simulink model "AckermanSimu"  (R2022a)
settings: Solver=VariableStepAuto  StartTime=0.0  StopTime=100  RelTol=1e-3
values from neighbouring files (symbols this model uses):
  a1 = 0.178    [param_tanques.m]
  A1 = 15.518    [param_tanques.m]
  A2 = A1 + 3e-5    (= 15.51803)    [param_tanques.m]
  a2 = a1+5e-5    (= 0.17805)    [param_tanques.m]
  g = 981    [param_tanques.m]
  K1 = K(1)    [Ackerman.m]    (also in param_tanques.m)
  K2 = [K(2) K(3)]    [Ackerman.m]    (also in param_tanques.m)
  Km = 4.6    [param_tanques.m]
  L0 = [0;0]    [param_tanques.m]
settings Model: Creator=joaom  LastModifiedBy=joaom

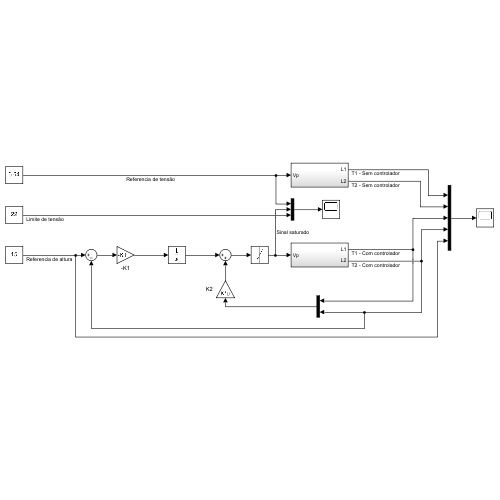
[thumbnail: Simulink's stored preview of the top-level diagram]
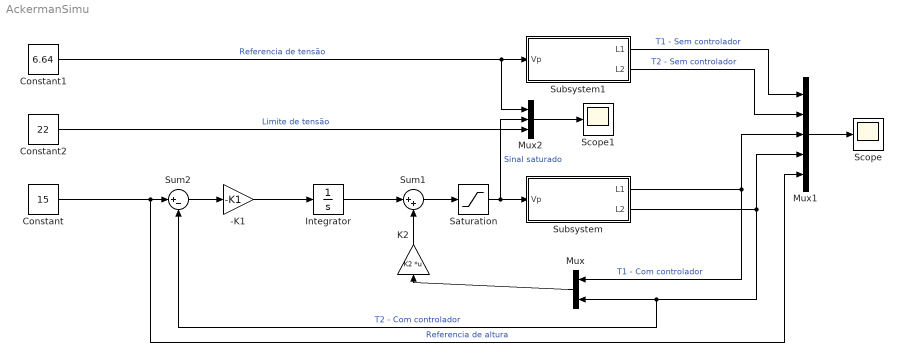
== system AckermanSimu ==
  -K1 : Gain  Gain=-K1
  Constant : Constant  Value=15
  Constant1 : Constant  Value=6.64
  Constant2 : Constant  Value=22
  Integrator : Integrator
  K2 : Gain  Gain=K2  Multiplication=Matrix(K*u)
  Mux : Mux  Inputs=2
  Mux1 : Mux  Inputs=5
  Mux2 : Mux  Inputs=3
  Saturation : Saturate  UpperLimit=22  LowerLimit=-22
  Scope : Scope
  Scope1 : Scope
  Subsystem : Subsystem
  Subsystem1 : Subsystem
  Sum1 : Sum  Inputs=|++
  Sum2 : Sum  Inputs=|+-
  wires:
  Constant/1 -> Mux1/5, Sum2/1  "Referencia de altura"
  Sum2/1 -> -K1/1
  -K1/1 -> Integrator/1
  Integrator/1 -> Sum1/1
  K2/1 -> Sum1/2
  Mux/1 -> K2/1
  Subsystem/2(L2) -> Mux1/4, Sum2/2, Mux/2  "T2 - Com controlador"
  Subsystem/1(L1) -> Mux1/3, Mux/1  "T1 - Com controlador"
  Mux1/1 -> Scope/1
  Constant1/1 -> Mux2/1, Subsystem1/1(Vp)  "Referencia de tensão"
  Subsystem1/1(L1) -> Mux1/1  "T1 - Sem controlador"
  Subsystem1/2(L2) -> Mux1/2  "T2 - Sem controlador"
  Mux2/1 -> Scope1/1
  Saturation/1 -> Mux2/2, Subsystem/1(Vp)  "Sinal saturado"
  Sum1/1 -> Saturation/1
  Constant2/1 -> Mux2/3  "Limite de tensão"

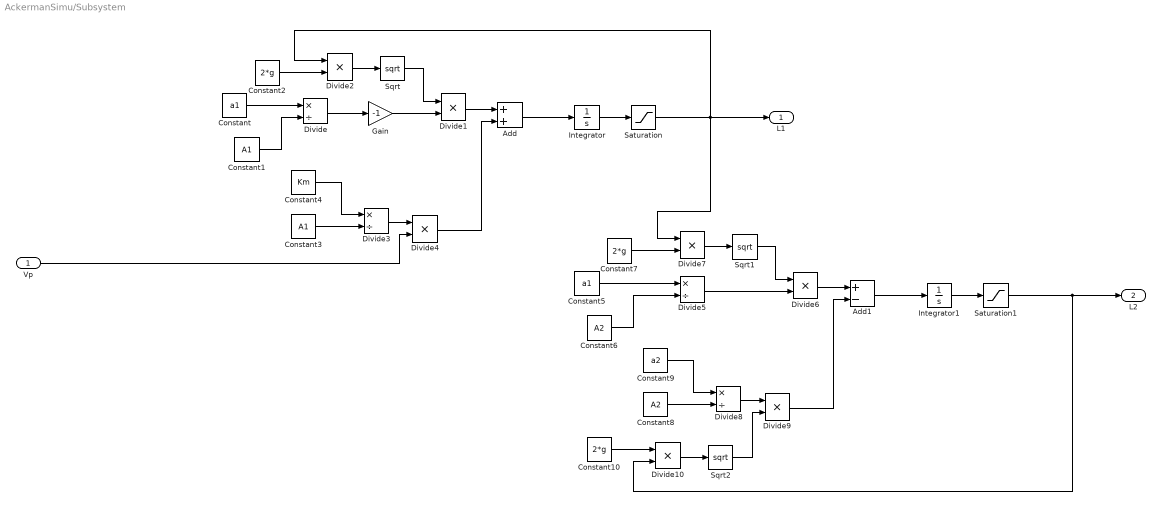
== system AckermanSimu/Subsystem ==
  Vp : Inport
  Add : Sum
  Add1 : Sum  Inputs=+-
  Constant : Constant  Value=a1
  Constant1 : Constant  Value=A1
  Constant10 : Constant  Value=2*g
  Constant2 : Constant  Value=2*g
  Constant3 : Constant  Value=A1
  Constant4 : Constant  Value=Km
  Constant5 : Constant  Value=a1
  Constant6 : Constant  Value=A2
  Constant7 : Constant  Value=2*g
  Constant8 : Constant  Value=A2
  Constant9 : Constant  Value=a2
  Divide{,3,5,8} (4 alike) : Product  Inputs=*/
  Divide{1..2,4,6..7,9..10} (7 alike) : Product  Inputs=**
  Gain : Gain  Gain=-1
  Integrator : Integrator  InitialCondition=L0(1)
  Integrator1 : Integrator  InitialCondition=L0(1)
  Saturation : Saturate  UpperLimit=30  LowerLimit=0
  Saturation1 : Saturate  UpperLimit=30  LowerLimit=0
  Sqrt : Sqrt
  Sqrt1 : Sqrt
  Sqrt2 : Sqrt
  L1 : Outport
  L2 : Outport  Port=2
  wires:
  Constant/1 -> Divide/1
  Constant1/1 -> Divide/2
  Divide/1 -> Gain/1
  Gain/1 -> Divide1/2
  Sqrt/1 -> Divide1/1
  Divide2/1 -> Sqrt/1
  Constant2/1 -> Divide2/2
  Divide1/1 -> Add/1
  Constant3/1 -> Divide3/2
  Constant4/1 -> Divide3/1
  Divide3/1 -> Divide4/1
  Vp/1 -> Divide4/2
  Divide4/1 -> Add/2
  Add/1 -> Integrator/1
  Integrator/1 -> Saturation/1
  Saturation/1 -> Divide2/1, Divide7/1, L1/1
  Constant5/1 -> Divide5/1
  Constant6/1 -> Divide5/2
  Divide5/1 -> Divide6/2
  Sqrt1/1 -> Divide6/1
  Divide7/1 -> Sqrt1/1
  Constant7/1 -> Divide7/2
  Divide6/1 -> Add1/1
  Constant8/1 -> Divide8/2
  Constant9/1 -> Divide8/1
  Divide8/1 -> Divide9/1
  Divide9/1 -> Add1/2
  Add1/1 -> Integrator1/1
  Integrator1/1 -> Saturation1/1
  Saturation1/1 -> Divide10/2, L2/1
  Constant10/1 -> Divide10/1
  Divide10/1 -> Sqrt2/1
  Sqrt2/1 -> Divide9/2

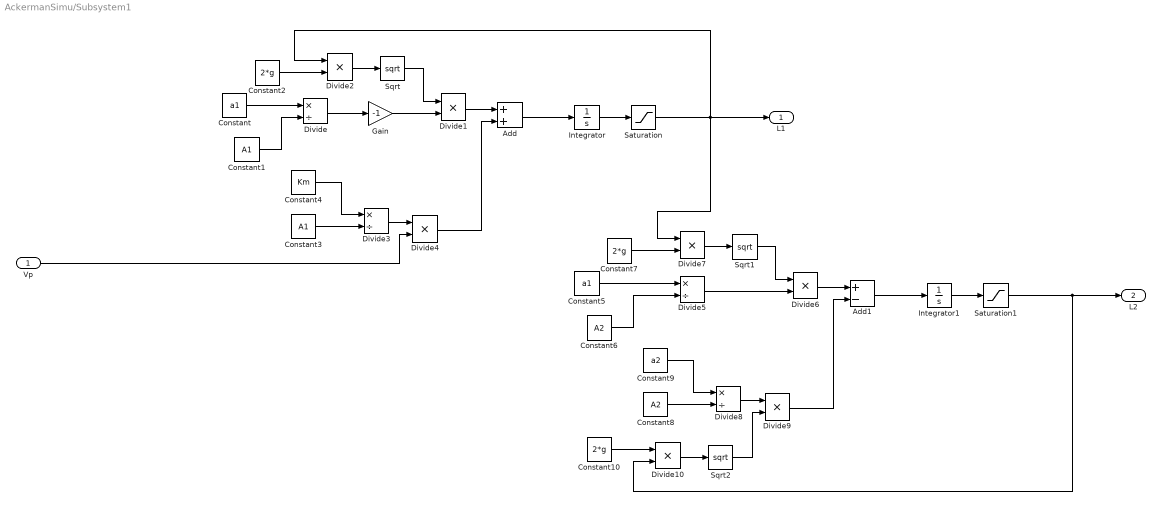
== system AckermanSimu/Subsystem1 ==
  Vp : Inport
  Add : Sum
  Add1 : Sum  Inputs=+-
  Constant : Constant  Value=a1
  Constant1 : Constant  Value=A1
  Constant10 : Constant  Value=2*g
  Constant2 : Constant  Value=2*g
  Constant3 : Constant  Value=A1
  Constant4 : Constant  Value=Km
  Constant5 : Constant  Value=a1
  Constant6 : Constant  Value=A2
  Constant7 : Constant  Value=2*g
  Constant8 : Constant  Value=A2
  Constant9 : Constant  Value=a2
  Divide{,3,5,8} (4 alike) : Product  Inputs=*/
  Divide{1..2,4,6..7,9..10} (7 alike) : Product  Inputs=**
  Gain : Gain  Gain=-1
  Integrator : Integrator  InitialCondition=L0(1)
  Integrator1 : Integrator  InitialCondition=L0(1)
  Saturation : Saturate  UpperLimit=30  LowerLimit=0
  Saturation1 : Saturate  UpperLimit=30  LowerLimit=0
  Sqrt : Sqrt
  Sqrt1 : Sqrt
  Sqrt2 : Sqrt
  L1 : Outport
  L2 : Outport  Port=2
  wires:
  Constant/1 -> Divide/1
  Constant1/1 -> Divide/2
  Divide/1 -> Gain/1
  Gain/1 -> Divide1/2
  Sqrt/1 -> Divide1/1
  Divide2/1 -> Sqrt/1
  Constant2/1 -> Divide2/2
  Divide1/1 -> Add/1
  Constant3/1 -> Divide3/2
  Constant4/1 -> Divide3/1
  Divide3/1 -> Divide4/1
  Vp/1 -> Divide4/2
  Divide4/1 -> Add/2
  Add/1 -> Integrator/1
  Integrator/1 -> Saturation/1
  Saturation/1 -> Divide2/1, Divide7/1, L1/1
  Constant5/1 -> Divide5/1
  Constant6/1 -> Divide5/2
  Divide5/1 -> Divide6/2
  Sqrt1/1 -> Divide6/1
  Divide7/1 -> Sqrt1/1
  Constant7/1 -> Divide7/2
  Divide6/1 -> Add1/1
  Constant8/1 -> Divide8/2
  Constant9/1 -> Divide8/1
  Divide8/1 -> Divide9/1
  Divide9/1 -> Add1/2
  Add1/1 -> Integrator1/1
  Integrator1/1 -> Saturation1/1
  Saturation1/1 -> Divide10/2, L2/1
  Constant10/1 -> Divide10/1
  Divide10/1 -> Sqrt2/1
  Sqrt2/1 -> Divide9/2
